simulink model "NonlinearModelSimulink_2016B_v2"  (R2016b)
settings: Solver=VariableStepAuto  StartTime=0.0  StopTime=30  RelTol=1e-3
InitFcn:
  | dynrotpend
undefined symbols (not defined in the file or in its folder): matrcomp, par
libraries: dspinverses x1
settings Model: Creator=jannekeblok  LastModifiedBy=janneke

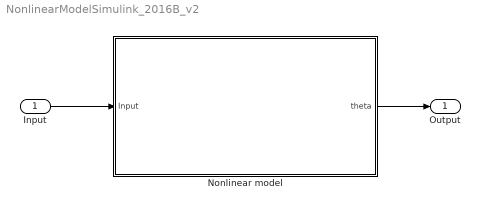
== system NonlinearModelSimulink_2016B_v2 ==
  Input : Inport
  Nonlinear model : Subsystem
  Output : Outport
  wires:
  Input/1 -> Nonlinear model/1("Input ")
  Nonlinear model/1(theta) -> Output/1

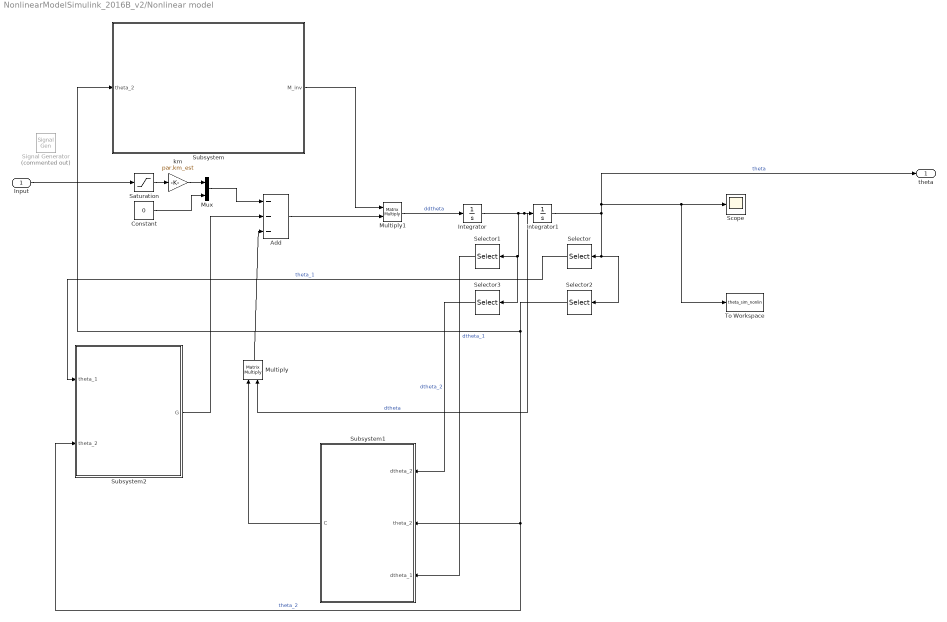
== system NonlinearModelSimulink_2016B_v2/Nonlinear model ==
  "Input " : Inport
  Add : Sum  Inputs=---
  Constant : Constant  Value=0
  Integrator : Integrator  InitialCondition=[0;0]
  Integrator1 : Integrator  InitialCondition=[pi;0]
  Multiply : Product  Multiplication=Matrix(*)
  Multiply1 : Product  Multiplication=Matrix(*)
  Mux : Mux  Inputs=2
  Saturation : Saturate  UpperLimit=1  LowerLimit=-1
  Scope : Scope
  Selector : Selector  InputPortWidth=2  IndexOptions=Index vector (dialog)  Indices=[1]  OutputSizes=1
  Selector1 : Selector  InputPortWidth=2  IndexOptions=Index vector (dialog)  Indices=[1]  OutputSizes=1
  Selector2 : Selector  InputPortWidth=2  IndexOptions=Index vector (dialog)  Indices=[2]  OutputSizes=1
  Selector3 : Selector  InputPortWidth=2  IndexOptions=Index vector (dialog)  Indices=[2]  OutputSizes=1
  Signal Generator : SignalGenerator  Commented=on  WaveForm=square  Amplitude=0.3
  Subsystem : Subsystem
  Subsystem1 : Subsystem
  Subsystem2 : Subsystem
  To Workspace : ToWorkspace  VariableName=theta_sim_nonlin  SaveFormat=Timeseries  SampleTime=-1
  km : Gain  Gain=par.km_est
  theta : Outport
  wires:
  Saturation/1 -> km/1
  Multiply/1 -> Add/3
  Subsystem2/1(G) -> Add/2
  Constant/1 -> Mux/2
  km/1 -> Mux/1
  Selector/1 -> Subsystem2/1(theta_1)  "theta_1"
  Subsystem/1(M_inv) -> Multiply1/1
  Subsystem1/1(C) -> Multiply/1
  Multiply1/1 -> Integrator/1  "ddtheta"
  Selector2/1 -> Subsystem2/2("theta_2 "), Subsystem1/2(theta_2), Subsystem/1("theta_2 ")  "theta_2"
  Add/1 -> Multiply1/2
  Mux/1 -> Add/1
  Selector1/1 -> Subsystem1/3(dtheta_1)  "dtheta_1"
  Integrator1/1 -> theta/1, To Workspace/1, Scope/1, Selector2/1, Selector/1  "theta"
  Selector3/1 -> Subsystem1/1(dtheta_2)  "dtheta_2"
  Integrator/1 -> Multiply/2, Integrator1/1, Selector1/1, Selector3/1  "dtheta"
  "Input "/1 -> Saturation/1

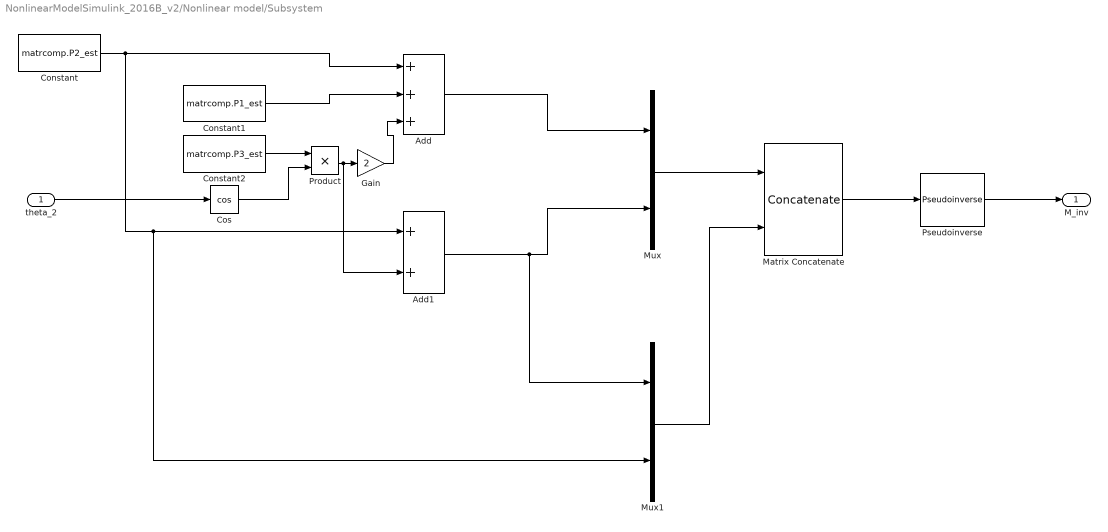
== system NonlinearModelSimulink_2016B_v2/Nonlinear model/Subsystem ==
  "theta_2 " : Inport
  Add : Sum  Inputs=+++
  Add1 : Sum
  Constant : Constant  Value=matrcomp.P2_est
  Constant1 : Constant  Value=matrcomp.P1_est
  Constant2 : Constant  Value=matrcomp.P3_est
  Cos : Trigonometry  Operator=cos
  Gain : Gain  Gain=2
  Matrix Concatenate : Concatenate  Mode=Multidimensional array  ConcatenateDimension=2
  Mux : Mux  Inputs=2
  Mux1 : Mux  Inputs=2
  Product : Product
  Pseudoinverse : dspinverses/Pseudoinverse  wanterr=off  SimulateUsing=Interpreted execution
  M_inv : Outport
  wires:
  Product/1 -> Add1/2, Gain/1
  Mux/1 -> Matrix Concatenate/1
  Cos/1 -> Product/2
  "theta_2 "/1 -> Cos/1
  Gain/1 -> Add/3
  Constant1/1 -> Add/2
  Constant2/1 -> Product/1
  Mux1/1 -> Matrix Concatenate/2
  Matrix Concatenate/1 -> Pseudoinverse/1
  Pseudoinverse/1 -> M_inv/1
  Add/1 -> Mux/1
  Add1/1 -> Mux/2, Mux1/1
  Constant/1 -> Mux1/2, Add1/1, Add/1

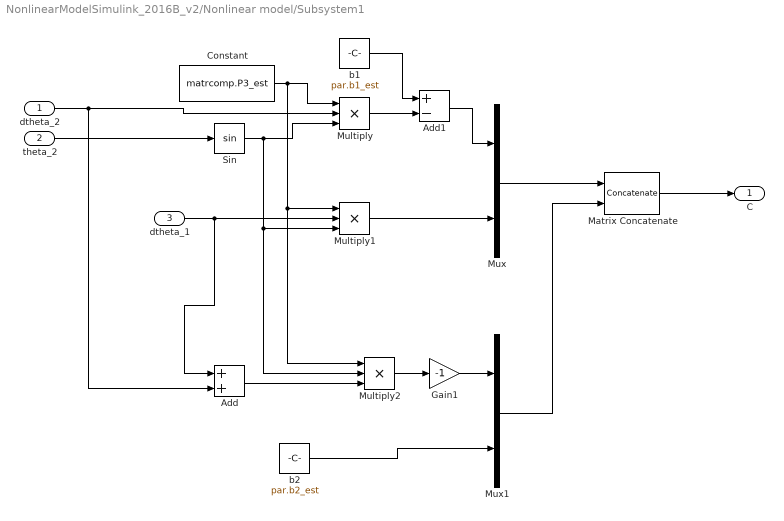
== system NonlinearModelSimulink_2016B_v2/Nonlinear model/Subsystem1 ==
  dtheta_2 : Inport
  theta_2 : Inport  Port=2
  dtheta_1 : Inport  Port=3
  Add : Sum
  Add1 : Sum  Inputs=+-
  Constant : Constant  Value=matrcomp.P3_est
  Gain1 : Gain  Gain=-1
  Matrix Concatenate : Concatenate  Mode=Multidimensional array  ConcatenateDimension=2
  Multiply : Product  Inputs=3
  Multiply1 : Product  Inputs=3
  Multiply2 : Product  Inputs=3
  Mux : Mux  Inputs=2
  Mux1 : Mux  Inputs=2
  Sin : Trigonometry
  b1 : Constant  Value=par.b1_est
  b2 : Constant  Value=par.b2_est
  C : Outport
  wires:
  Gain1/1 -> Mux1/1
  Mux1/1 -> Matrix Concatenate/2
  Add/1 -> Multiply2/3
  Multiply2/1 -> Gain1/1
  dtheta_1/1 -> Add/1, Multiply1/2
  Multiply/1 -> Add1/2
  Matrix Concatenate/1 -> C/1
  Multiply1/1 -> Mux/2
  Constant/1 -> Multiply1/1, Multiply2/1, Multiply/1
  Mux/1 -> Matrix Concatenate/1
  b2/1 -> Mux1/2
  dtheta_2/1 -> Add/2, Multiply/2
  theta_2/1 -> Sin/1
  Sin/1 -> Multiply1/3, Multiply2/2, Multiply/3
  Add1/1 -> Mux/1
  b1/1 -> Add1/1

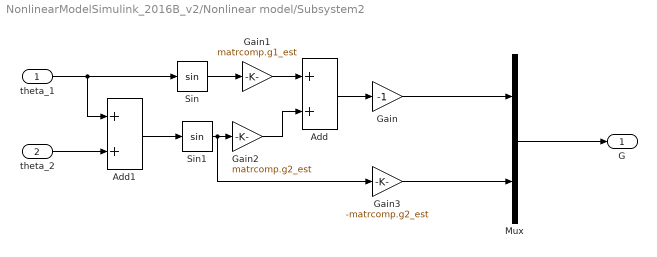
== system NonlinearModelSimulink_2016B_v2/Nonlinear model/Subsystem2 ==
  theta_1 : Inport
  "theta_2 " : Inport  Port=2
  Add : Sum
  Add1 : Sum
  Gain : Gain  Gain=-1
  Gain1 : Gain  Gain=matrcomp.g1_est
  Gain2 : Gain  Gain=matrcomp.g2_est
  Gain3 : Gain  Gain=-matrcomp.g2_est
  Mux : Mux  Inputs=2
  Sin : Trigonometry
  Sin1 : Trigonometry
  G : Outport
  wires:
  Gain2/1 -> Add/2
  Mux/1 -> G/1
  Add1/1 -> Sin1/1
  Gain3/1 -> Mux/2
  Add/1 -> Gain/1
  Sin/1 -> Gain1/1
  Sin1/1 -> Gain3/1, Gain2/1
  Gain1/1 -> Add/1
  Gain/1 -> Mux/1
  "theta_2 "/1 -> Add1/2
  theta_1/1 -> Sin/1, Add1/1
